simulink library "Test_lib"  (R2023b)
settings: Solver=VariableStepAuto  StartTime=0.0  StopTime=10.0  RelTol=1e-3
undefined symbols (not defined in the file): Spline_Num_Poses_default, Spline_Ref_Poses_default
settings Model: Creator=FIRSTMentor  LastModifiedBy=ander

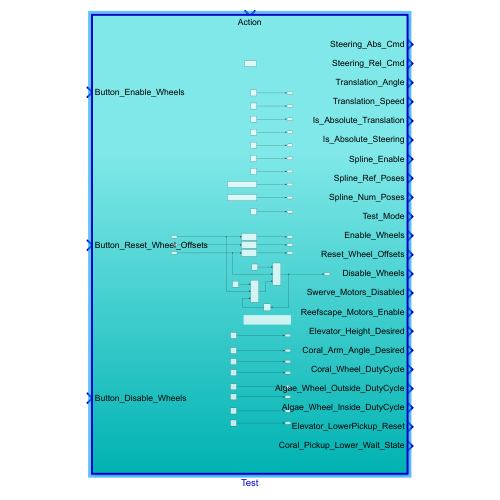
[thumbnail: Simulink's stored preview of the top-level diagram]
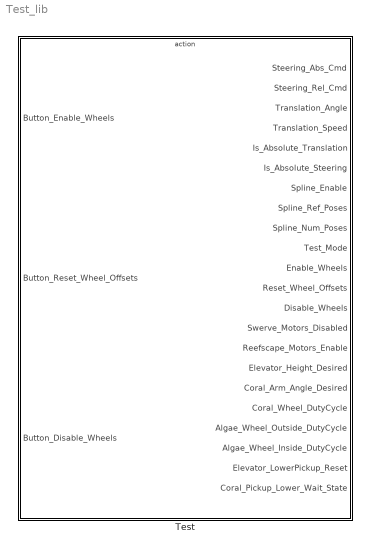
== system Test_lib ==
  Test : Subsystem  TreatAsAtomicUnit=on

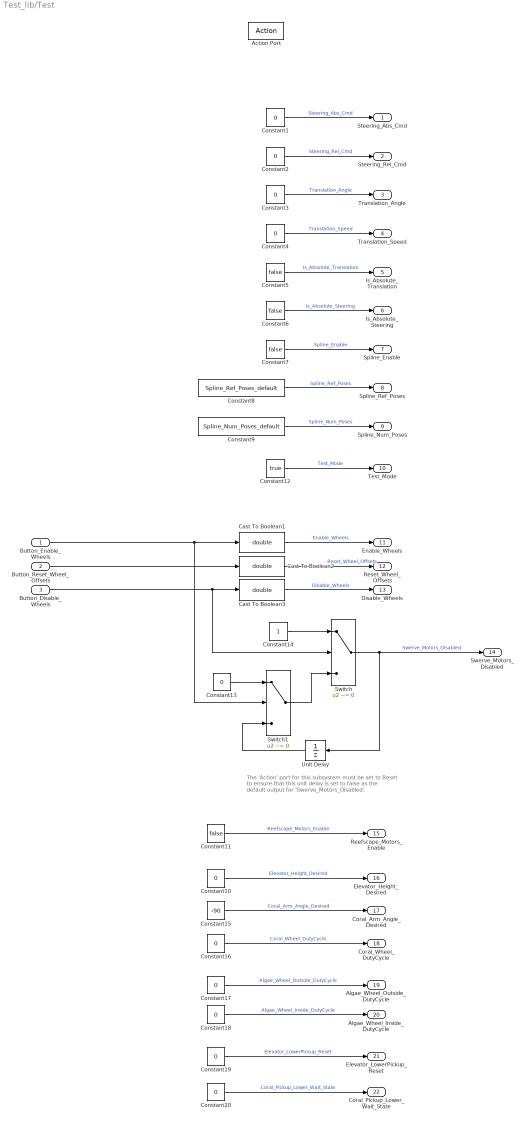
== system Test_lib/Test ==
  note: The 'Action' port for this subsystem must be set to Reset to ensure that this unit delay is set to false as the default output for 'Swerve_Motors_Disabled'.
  Button_Enable_Wheels : Inport
  Button_Reset_Wheel_Offsets : Inport  Port=2
  Button_Disable_Wheels : Inport  Port=3
  Action Port : ActionPort  InitializeStates=reset
  Cast To Boolean1 : DataTypeConversion  OutDataTypeStr=double  SaturateOnIntegerOverflow=off  RndMeth=Floor
  Cast To Boolean2 : DataTypeConversion  OutDataTypeStr=double  SaturateOnIntegerOverflow=off  RndMeth=Floor
  Cast To Boolean3 : DataTypeConversion  OutDataTypeStr=double  SaturateOnIntegerOverflow=off  RndMeth=Floor
  Constant{1..4,10,13,16..18} (9 alike) : Constant  Value=0
  Constant11 : Constant  Value=false  OutDataTypeStr=boolean
  Constant12 : Constant  Value=true  OutDataTypeStr=boolean
  Constant14 : Constant
  Constant15 : Constant  Value=-90
  Constant19 : Constant  Value=0  OutDataTypeStr=boolean
  Constant20 : Constant  Value=0  OutDataTypeStr=boolean
  Constant5 : Constant  Value=false
  Constant6 : Constant  Value=false
  Constant7 : Constant  Value=false  OutDataTypeStr=boolean
  Constant8 : Constant  Value=Spline_Ref_Poses_default
  Constant9 : Constant  Value=Spline_Num_Poses_default  OutDataTypeStr=double
  Switch : Switch  Criteria=u2 ~= 0  SaturateOnIntegerOverflow=off  InputSameDT=off
  Switch1 : Switch  Criteria=u2 ~= 0  SaturateOnIntegerOverflow=off  InputSameDT=off
  Unit Delay : UnitDelay  SampleTime=-1  HasFrameUpgradeWarning=on
  Steering_Abs_Cmd : Outport
  Steering_Rel_Cmd : Outport  Port=2
  Translation_Angle : Outport  Port=3
  Translation_Speed : Outport  Port=4
  Is_Absolute_Translation : Outport  Port=5
  Is_Absolute_Steering : Outport  Port=6
  Spline_Enable : Outport  Port=7
  Spline_Ref_Poses : Outport  Port=8
  Spline_Num_Poses : Outport  Port=9
  Test_Mode : Outport  Port=10
  Enable_Wheels : Outport  Port=11
  Reset_Wheel_Offsets : Outport  Port=12
  Disable_Wheels : Outport  Port=13
  Swerve_Motors_Disabled : Outport  Port=14
  Reefscape_Motors_Enable : Outport  Port=15
  Elevator_Height_Desired : Outport  Port=16
  Coral_Arm_Angle_Desired : Outport  Port=17
  Coral_Wheel_DutyCycle : Outport  Port=18
  Algae_Wheel_Outside_DutyCycle : Outport  Port=19
  Algae_Wheel_Inside_DutyCycle : Outport  Port=20
  Elevator_LowerPickup_Reset : Outport  Port=21
  Coral_Pickup_Lower_Wait_State : Outport  Port=22
  wires:
  Constant6/1 -> Is_Absolute_Steering/1  "Is_Absolute_Steering"
  Constant4/1 -> Translation_Speed/1  "Translation_Speed"
  Constant5/1 -> Is_Absolute_Translation/1  "Is_Absolute_Translation"
  Constant3/1 -> Translation_Angle/1  "Translation_Angle"
  Constant2/1 -> Steering_Rel_Cmd/1  "Steering_Rel_Cmd"
  Constant1/1 -> Steering_Abs_Cmd/1  "Steering_Abs_Cmd"
  Constant7/1 -> Spline_Enable/1  "Spline_Enable"
  Constant9/1 -> Spline_Num_Poses/1  "Spline_Num_Poses"
  Constant8/1 -> Spline_Ref_Poses/1  "Spline_Ref_Poses"
  Constant12/1 -> Test_Mode/1  "Test_Mode"
  Button_Reset_Wheel_Offsets/1 -> Cast To Boolean2/1
  Button_Disable_Wheels/1 -> Cast To Boolean3/1, Switch/2
  Cast To Boolean2/1 -> Reset_Wheel_Offsets/1  "Reset_Wheel_Offsets"
  Cast To Boolean3/1 -> Disable_Wheels/1  "Disable_Wheels"
  Switch/1 -> Swerve_Motors_Disabled/1, Unit Delay/1  "Swerve_Motors_Disabled"
  Button_Enable_Wheels/1 -> Cast To Boolean1/1, Switch1/2
  Unit Delay/1 -> Switch1/3
  Constant13/1 -> Switch1/1
  Constant14/1 -> Switch/1
  Switch1/1 -> Switch/3
  Cast To Boolean1/1 -> Enable_Wheels/1  "Enable_Wheels"
  Constant10/1 -> Elevator_Height_Desired/1  "Elevator_Height_Desired"
  Constant11/1 -> Reefscape_Motors_Enable/1  "Reefscape_Motors_Enable"
  Constant15/1 -> Coral_Arm_Angle_Desired/1  "Coral_Arm_Angle_Desired"
  Constant16/1 -> Coral_Wheel_DutyCycle/1  "Coral_Wheel_DutyCycle"
  Constant17/1 -> Algae_Wheel_Outside_DutyCycle/1  "Algae_Wheel_Outside_DutyCycle"
  Constant18/1 -> Algae_Wheel_Inside_DutyCycle/1  "Algae_Wheel_Inside_DutyCycle"
  Constant19/1 -> Elevator_LowerPickup_Reset/1  "Elevator_LowerPickup_Reset"
  Constant20/1 -> Coral_Pickup_Lower_Wait_State/1  "Coral_Pickup_Lower_Wait_State"
